simulink model "boost_CM_averaged"  (Simulink 6.5)
settings: Solver=ode45  StartTime=0.0  StopTime=2/60  MaxStep=10e-6  RelTol=1e-3
settings Model: Creator=Mama  LastModifiedBy=Dragan Maksimovic
settings DebuggingCC: AlgebraicLoopMsg=none  SolverPrmCheckMsg=none  UnconnectedOutputMsg=none

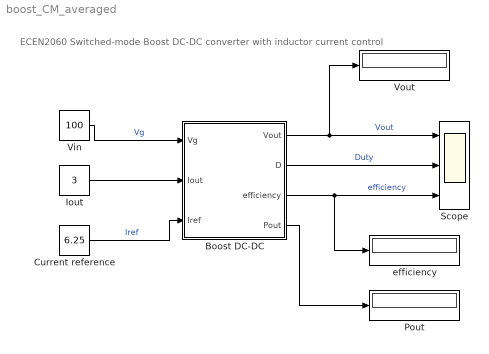
== system boost_CM_averaged ==
  note: ECEN2060
      | Switched-mode Boost
      | DC-DC converter
      | with inductor current control
  Boost DC-DC : Subsystem  mask{C=10e-6, Vo=200, RL=0.5, IQ=0.03}
      mask prompts: C "Capacitance"; Vo "Initial capacitor voltage"; RL "Input port series resistance"; IQ "Switching loss current"
      mask help: Averaged model of a boost (step-up) DC-DC converter with input current control. Model includes losses due to input port resistance RL and output-port switching-loss current Isw.
      mask Display:
      | text(0.5,0.9,'Boost','horizontalAlignment', 'center');
      | text(0.5,0.8,'DC-DC','horizontalAlignment', 'center');
      | text(0.5,0.7,'(averaged, C)','horizontalAlignment', 'center');
      | text(0.5,0.6,'current control','horizontalAlignment', 'center');
  Current reference : Constant  Value=6.25  OutDataType=sfix(16)  ConRadixGroup=Use specified scaling  OutScaling=2^0  SampleTime=inf  FramePeriod=inf
  Iout : Constant  Value=3  OutDataType=sfix(16)  ConRadixGroup=Use specified scaling  OutScaling=2^0  SampleTime=inf  FramePeriod=inf
  Pout : Display
  Scope : Scope  NumInputPorts=3
      settings: TimeRange=0.035  YMin=199.8~0.5152~0.95915  YMax=200~0.516~0.9591599999999999
  Vin : Constant  Value=100  OutDataType=sfix(16)  ConRadixGroup=Use specified scaling  OutScaling=2^0  SampleTime=inf  FramePeriod=inf
  Vout : Display
  efficiency : Display
  wires:
  Current reference/1 -> Boost DC-DC/3(Iref)  "Iref"
  Vin/1 -> Boost DC-DC/1(Vg)  "Vg"
  Boost DC-DC/1(Vout) -> Vout/1, Scope/1  "Vout"
  Boost DC-DC/2(D) -> Scope/2  "Duty"
  Boost DC-DC/3(efficiency) -> Scope/3, efficiency/1  "efficiency"
  Boost DC-DC/4(Pout) -> Pout/1
  Iout/1 -> Boost DC-DC/2(Iout)

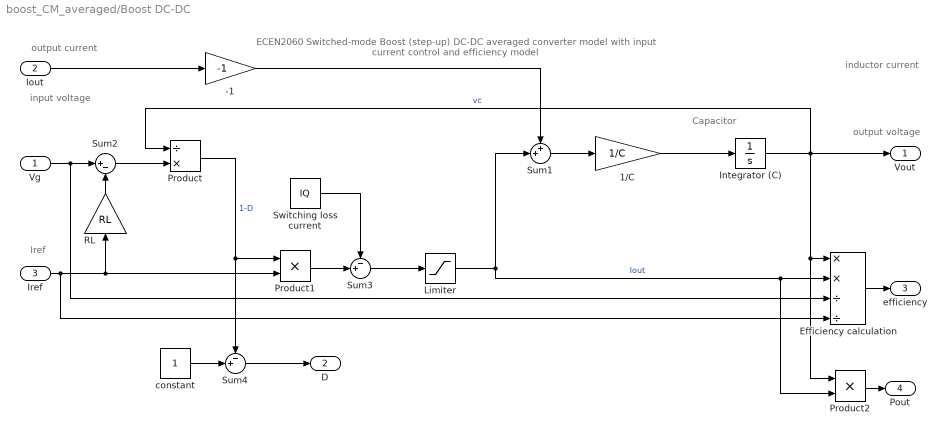
== system boost_CM_averaged/Boost DC-DC ==
  note: ECEN2060 Switched-mode Boost (step-up) DC-DC averaged converter model
      | with input current control and efficiency model
  note: output voltage
  note: inductor current
  note: output current
  note: input voltage
  note: Iref
  note: Capacitor
  Vg : Inport
  Iout : Inport  Port=2
  Iref : Inport  Port=3
  -1 : Gain  Gain=-1
  1/C : Gain  Gain=1/C
  Efficiency calculation : Product  Inputs=**//  RndMeth=Zero
  Integrator (C) : Integrator  InitialCondition=Vo
  Limiter : Saturate  UpperLimit=inf  LowerLimit=0
  Product : Product  Inputs=/*  RndMeth=Zero
  Product1 : Product  Inputs=**  RndMeth=Zero
  Product2 : Product  Inputs=**  RndMeth=Zero
  RL : Gain  Orientation=up  Gain=RL
  Sum1 : Sum  Inputs=++|
  Sum2 : Sum  Inputs=|+-
  Sum3 : Sum  Inputs=-+|
  Sum4 : Sum  Inputs=-+|
  Switching loss current : Constant  Value=IQ  OutDataType=sfix(16)  ConRadixGroup=Use specified scaling  OutScaling=2^0  SampleTime=inf  FramePeriod=inf
  constant : Constant  Value=1  OutDataType=sfix(16)  ConRadixGroup=Use specified scaling  OutScaling=2^0  SampleTime=inf  FramePeriod=inf
  Vout : Outport
  D : Outport  Port=2
  efficiency : Outport  Port=3
  Pout : Outport  Port=4
  wires:
  Sum1/1 -> 1/C/1
  1/C/1 -> Integrator (C)/1
  Integrator (C)/1 -> Vout/1, Product/1, Efficiency calculation/1, Product2/1  "vc"
  Iout/1 -> -1/1
  -1/1 -> Sum1/1
  RL/1 -> Sum2/2
  Iref/1 -> RL/1, Product1/2, Efficiency calculation/4
  Vg/1 -> Sum2/1, Efficiency calculation/3
  Sum2/1 -> Product/2
  Product/1 -> Product1/1, Sum4/1  "1-D"
  Product1/1 -> Sum3/2
  Switching loss current/1 -> Sum3/1
  Sum3/1 -> Limiter/1
  Limiter/1 -> Sum1/2, Efficiency calculation/2, Product2/2  "Iout"
  Efficiency calculation/1 -> efficiency/1
  constant/1 -> Sum4/2
  Sum4/1 -> D/1
  Product2/1 -> Pout/1
